simulink model "LandingGearMode_sfunction"  (R2015a)
settings: Solver=FixedStepDiscrete  StartTime=0.0  StopTime=10.0  FixedStep=0.2  RelTol=1e-3
PreLoadFcn:
  | load busdata;
settings Model: RequirementInfo={'other' '..\requirements\DisplaySystemRequirements.docx' '@Simulink_requirement_item_36' 'true' 'Landing Gear' '' } %GIDa_b67bee78_da89_4e0d_9cae_24e8ea5a1e59  CovPath=LandingGearModes  CovMetricSettings=dcmw  CovHTMLOptions=-sRT=1 -aTS=1 -bRG=1 -bTC=1 -hTR=0 -nFC=0 -scm=1 -bcm=1 -xEv=0  CovModelRefEnable=off  Creator=siddhars  LastModifiedBy=syoon
settings OptimizationCC: BlockReduction=off  InlineParams=on  UseDivisionForNetSlopeComputation=on  ExpressionDepthLimit=2147483647  EfficientFloat2IntCast=on  OptimizeModelRefInitCode=on
settings DebuggingCC: SignalInfNanChecking=error  SignalRangeChecking=error  ReadBeforeWriteMsg=EnableAllAsError  WriteAfterWriteMsg=EnableAllAsError  WriteAfterReadMsg=EnableAllAsError  AlgebraicLoopMsg=error  ArtificialAlgebraicLoopMsg=error  SaveWithDisabledLinksMsg=error  SaveWithParameterizedLinksMsg=error  BlockPriorityViolationMsg=error  SolverPrmCheckMsg=error  InheritedTsInSrcMsg=error  DiscreteInheritContinuousMsg=error  SigSpecEnsureSampleTimeMsg=error  CheckMatrixSingularityMsg=error  IntegerOverflowMsg=error  ParameterUnderflowMsg=error  ParameterPrecisionLossMsg=error  ParameterTunabilityLossMsg=error  UnderSpecifiedDataTypeMsg=error  UnnecessaryDatatypeConvMsg=warning  VectorMatrixConversionMsg=error  SignalLabelMismatchMsg=error  UnconnectedInputMsg=error  UnconnectedOutputMsg=error  UnconnectedLineMsg=error  SFcnCompatibilityMsg=error  BusObjectLabelMismatch=error  RootOutportRequireBusObject=error  ModelReferenceIOMsg=error  ModelReferenceIOMismatchMessage=error  UnknownTsInhSupMsg=error  ModelReferenceDataLoggingMessage=error  StateNameClashWarn=warning  StrictBusMsg=ErrorOnBusTreatedAsVector
settings HardwareCC: ProdIntDivRoundTo=Zero  ProdEndianess=LittleEndian  ProdHWDeviceType=Intel->x86/Pentium  TargetBitPerLong=64  TargetBitPerPointer=64  TargetIntDivRoundTo=Zero  TargetEndianess=LittleEndian  TargetWordSize=64  TargetHWDeviceType=Intel->x86-64
settings RTWCC: SystemTargetFile=ert.tlc  TemplateMakefile=ert_default_tmf  Description=Embedded Coder  GenerateReport=on  IncludeHyperlinkInReport=on  LaunchReport=on  PortableWordSizes=on  GenerateTraceInfo=on  GenerateTraceReport=on  GenerateTraceReportSl=on  GenerateTraceReportSf=on  GenerateTraceReportEml=on  GenerateCodeMetricsReport=on
settings CodeAppCC: ForceParamTrailComments=on  IgnoreCustomStorageClasses=off  MangleLength=4  CustomSymbolStrType=$N$R$M  ReqsInCode=on
settings ERTTargetCC: UtilityFuncGeneration=Shared location  ParMdlRefBuildCompliant=on  CompOptLevelCompliant=on  ConcurrentExecutionCompliant=on  IncludeMdlTerminateFcn=off  GeneratePreprocessorConditionals=Disable all  SuppressErrorStatus=on  ERTFirstTimeCompliant=on  SupportAbsoluteTime=off  SupportNonFinite=off  SupportComplex=off  SupportContinuousTime=off  SupportVariableSizeSignals=off  ParenthesesLevel=Maximum  CastingMode=Standards  ModelStepFunctionPrototypeControlCompliant=on  CPPClassGenCompliant=on  GenerateSharedConstants=off  ERTCustomFileTemplate=example_file_process.tlc  PreserveExpressionOrder=on  PreserveIfCondition=on  EnableSignedLeftShifts=off
settings ConfigComp: Description=Design Verifier Custom Configuration Component  DVModelCoverageObjectives=MCDC  DVMaxTestCaseSteps=500  DVTestSuiteOptimization=CombinedObjectives (Nonlinear Extended)  DVDetectActiveLogic=on  DVSaveHarnessModel=on  DVModelReferenceHarness=on

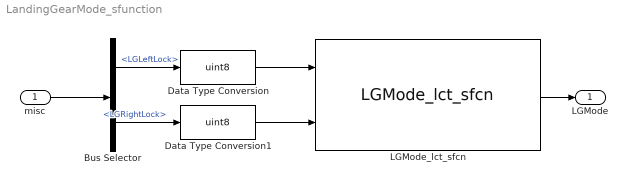
== system LandingGearMode_sfunction ==
  misc : Inport  RequirementInfo={'other' '..\requirements\DisplaySystemRequirements.docx' '@Simulink_requirement_item_33' 'true' 'The state of the landing gear will be contained in a bus object: MiscData. This bus object is defined as follows:' '' } %GIDa_a5b9fd2b_8586_4fb0_a66b_565a39eb0306  OutDataTypeStr=Bus: MiscData  PortDimensions=1  SampleTime=0.2
  Bus Selector : BusSelector  OutputSignals=LGLeftLock,LGRightLock
  Data Type Conversion : DataTypeConversion  OutDataTypeStr=uint8
  Data Type Conversion1 : DataTypeConversion  OutDataTypeStr=uint8
  LGMode_lct_sfcn : S-Function  FunctionName=LGMode_lct_sfcn  mask(Legacy Function){SFunctionSpec=double y1 = LGMode_lct(uint8 u1, uint8 u2), ShowSpec=on}
      mask prompts: ShowSpec "Display function specification"
      mask help:
      | This block allows you to call the legacy functions specified by the following Legacy Code Tool definition:
      | def.SFunctionName = 'LGMode_lct_sfcn';
      | def.OutputFcnSpec = 'double y1 = LGMode_lct(uint8 u1, uint8 u2)';
      | def.StartFcnSpec = 'void LandingGearMode_initialize(void)';
      | def.HeaderFiles = {'LGMode_lct.h'};
      | def.SourceFiles = {'LGMode_lct.c', 'LandingGearMode.c'};
      | def.IncPaths = {'..\src', '..\src\LandingGearMode_ert_rtw'};
      | def.SrcPaths = {'..\src', '..\src\LandingGearMode_ert_rtw'};
      | def.Options.supportCoverage = true;
      mask Help: <p>This block was generated automatically by the Legacy Code Tool. For detailed help on this tool, call<a href="matlab:legacy_code('help')"> legacy_code('help')</a>.</p>
      mask Callback ShowSpec:
      | if strcmp(get_param(gcbh, 'ShowSpec'), 'on')
      |   set_param(gcbh, 'MaskDisplay', sprintf('fprintf(''%s'');', get_param(gcbh, 'SFunctionSpec')));
      | else
      |   set_param(gcbh, 'MaskDisplay', sprintf('fprintf(''%s'');', get_param(gcbh, 'FunctionName')));
      | end
      mask Display: fprintf('double y1 = LGMode_lct(uint8 u1, uint8 u2)');
  LGMode : Outport  RequirementInfo={'other' '..\requirements\DisplaySystemRequirements.docx' '@Simulink_requirement_item_34' 'true' 'The output of the system shall be an integer of type double, LandingGearMode.' '' } %GIDa_59beb7db_0a03_418d_b1e3_a7a5af8dcfe0
  wires:
  LGMode_lct_sfcn/1 -> LGMode/1
  misc/1 -> Bus Selector/1
  Bus Selector/2 -> Data Type Conversion1/1  "<LGRightLock>"
  Bus Selector/1 -> Data Type Conversion/1  "<LGLeftLock>"
  Data Type Conversion/1 -> LGMode_lct_sfcn/1
  Data Type Conversion1/1 -> LGMode_lct_sfcn/2
